simulink model "statcom_completed"  (Simulink 8.7)
settings: Solver=ode45  StartTime=0.0  StopTime=0.5  RelTol=1e-3
undefined symbols (not defined in the file): D11, Delta
libraries: powerlib x16, powerlib_extras x3
settings Model: Creator=CPLAB_9  LastModifiedBy=Shahrukh
settings DataIOCC: SignalLoggingSaveFormat=ModelDataLogs
settings OptimizationCC: ExpressionDepthLimit=2147483647
settings DebuggingCC: SolverPrmCheckMsg=warning  FcnCallInpInsideContextMsg=UseLocalSettings  StateNameClashWarn=warning
settings GRTTargetCC: CombineOutputUpdateFcns=off  GRTInterface=on

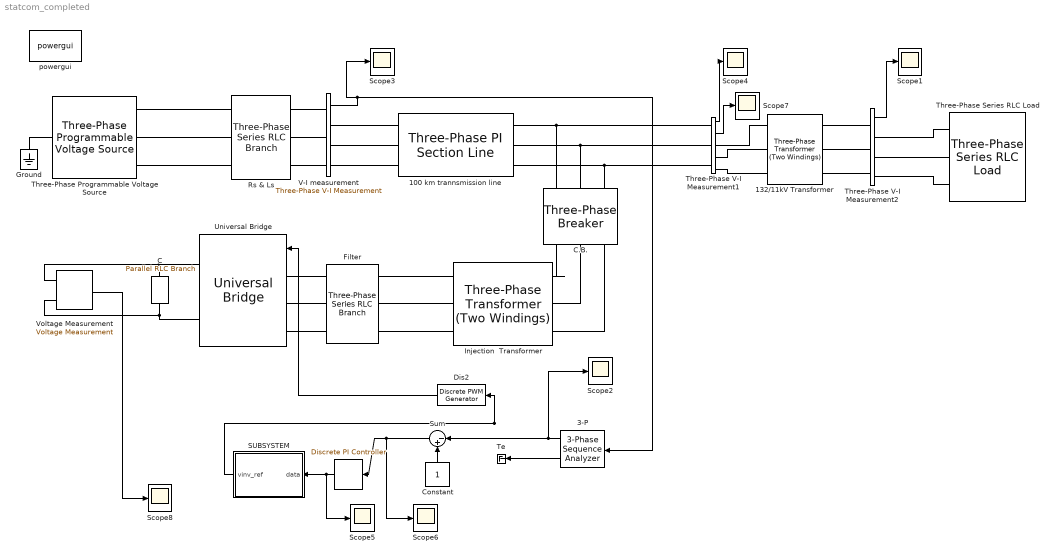
== system statcom_completed ==
  " " : powerlib_extras/Discrete  Control Blocks/Discrete PI Controller  Kp=0.5  Ki=500  Par_Limits=[1e6 -1e6]  Init=0  Ts=50e-6
  " 132/11kV Transformer" : powerlib/Elements/Three-Phase Transformer (Two Windings)  Winding1Connection=Delta (D11)  Winding2Connection=Delta (D11)  CoreType=Three single-phase transformers  SetSaturation=off  Hysteresis=off  DataFile='hysteresis'  SetInitialFlux=off  Measurements=None  UNITS=pu  NominalPower=[ 132e3 , 50 ]  Winding1="[ 132e3  , 0.01, 0.08 ]"  Winding2=[ 11e3 , 0.001, 0.008 ]  Rm=500  Lm=500  L0=0.5  Saturation=[ 0,0 ; 0.0024,1.2 ; 1.0,1.52 ]  InitialFluxes=[ 0.8 , -0.8 , 0.7 ]  MoreParameters=off  BreakLoop=off  DataType=off  TransfoNumber=1
  " Voltage Measurement" : powerlib/Measurements/Voltage Measurement  PhasorSimulation=off  OutputType=Complex  PSBequivalent=0
  "   C.B." : powerlib/Elements/Three-Phase Breaker  InitialState=open  SwitchA=on  SwitchB=on  SwitchC=on  SwitchTimes=[0.1 0.4]  External=off  BreakerResistance=0.01  SnubberResistance=1e5  SnubberCapacitance=inf  Measurements=Breaker voltages
  100 km trannsmission line : powerlib/Elements/Three-Phase PI Section Line  LConnTagsString=a|b|c  RConnTagsString=A|B|C  Frequency=50  Resistances=[ 0.00001 0.0001]  Inductances="[ 0.0000001e-3  0.0000001e-3]"  Capacitances=[0.00001e-9 0.000001e-9]  Length=100
  3-P : powerlib_extras/Measurements/3-Phase Sequence Analyzer  f1=50  n=1  seq=Positive
  C : powerlib/Elements/Parallel RLC Branch  LConnTagsString=a  RConnTagsString=__new0  BranchType=C  Resistance=[]  Inductance=[]  SetiL0=off  InitialCurrent=0  Capacitance=1000e-6  Setx0=off  InitialVoltage=600  Measurements=Branch voltage
  Constant : Constant
  Dis2 : powerlib_extras/Discrete  Control Blocks/Discrete PWM Generator  GeneratorMode="3-arm  bridge (6 pulses)"  Fc=5000  Ts=5e-6  Internal=off  mIndex=1  Freq=50  Phase=90
  Filter : powerlib/Elements/Three-Phase Series RLC Branch  LConnTagsString=A|B|C  RConnTagsString=A|B|C  BranchType=L  Resistance=0.001  Inductance=7.5  Capacitance=1.0  Measurements=Branch voltages
  Ground : powerlib/Elements/Ground  LConnTagsString=a
  Injection  Transformer : powerlib/Elements/Three-Phase Transformer (Two Windings)  Winding1Connection=Delta (D11)  Winding2Connection=Delta (D11)  CoreType=Three single-phase transformers  SetSaturation=off  Hysteresis=off  DataFile='hysteresis'  SetInitialFlux=off  Measurements=None  UNITS=pu  NominalPower=[ 132e3 , 50 ]  Winding1=[ 132e3 , 0.00002 , 0.00008 ]  Winding2=[ 11e3 , 0.00002 , 0.00008 ]  Rm=500  Lm=500  L0=0.5  Saturation=[ 0,0 ; 0.0024,1.2 ; 1.0,1.52 ]  InitialFluxes=[ 0.8 , -0.8 , 0.7 ]  MoreParameters=off  BreakLoop=off  DataType=off  TransfoNumber=1
  Rs & Ls : powerlib/Elements/Three-Phase Series RLC Branch  LConnTagsString=A|B|C  RConnTagsString=A|B|C  BranchType=RL  Resistance=0.02  Inductance=0.01  Capacitance=1.0  Measurements=Branch voltages
  SUBSYSTEM : Subsystem
  Scope{1..8} (8 alike) : Scope
  Sum : Sum  Inputs=|-+
  Te : Terminator
  Three-Phase Programmable Voltage Source : powerlib/Electrical Sources/Three-Phase Programmable Voltage Source  PositiveSequence="[132e3  0 50]"  VariationEntity=Amplitude  VariationType=Table of time-amplitude pairs  VariationTypeAlt=Step  VariationStep=0.5  VariationRate=10  VariationMagnitude=0.3  VariationFrequency=2  VariationTiming=[1 2]  VariationPhaseA=off  Amplitudes=[1 1.2 1 1]  TimeValues=[0 0.1 0.4 0.5]  HarmonicGeneration=off  HarmonicA=[3 0.2 -25 0]  HarmonicB=[2 0.15 35 2]  Timing="[0.05  3]"  BusType=swing  Pref=0  Qref=0  Qmin=-inf  Qmax=inf
  Three-Phase Series RLC Load : powerlib/Elements/Three-Phase Series RLC Load  LConnTagsString=A|B|C  Configuration=Y (grounded)  NominalVoltage=11e3  Vabc=[1e3 1e3 1e3]  Vabcp=[1e3 1e3 1e3]  NominalFrequency=50  UnbalancedPower=off  ActivePower=100e3  InductivePower=1000  CapacitivePower=1000  Pabc=[10e3 9e3 11e3]  QLabc=[100 90 110]  QCabc=[100 90 110]  Pabcp=[10e3 9e3 11e3]  QLabcp=[100 90 110]  QCabcp=[100 90 110]  Measurements=Branch voltages  LoadType=constant Z
  Three-Phase V-I Measurement1 : powerlib/Measurements/Three-Phase V-I Measurement  VoltageMeasurement=phase-to-ground  SetLabelV=off  LabelV=Vabc  Vpu=on  VpuLL=off  CurrentMeasurement=yes  SetLabelI=off  LabelI=Iabc  Ipu=off  Pbase=100e6  Vbase=132e3  OutputType=Complex  PhasorSimulation=off  PSBequivalent=0
  Three-Phase V-I Measurement2 : powerlib/Measurements/Three-Phase V-I Measurement  VoltageMeasurement=phase-to-phase  SetLabelV=off  LabelV=Vabc  Vpu=off  VpuLL=on  CurrentMeasurement=no  SetLabelI=off  LabelI=Iabc  Ipu=off  Pbase=100e6  Vbase=11e3  OutputType=Complex  PhasorSimulation=off  PSBequivalent=0
  Universal Bridge : powerlib/Power Electronics/Universal Bridge  Arms=3  SnubberResistance=1e5  SnubberCapacitance=inf  Device=IGBT / Diodes  Ron=1e-3  Lon=0  ForwardVoltages="[  0  0  ]"  ForwardVoltage=0  GTOparameters=[ 10e-6 , 20e-6 ]  IGBTparameters=[ 1e-6 , 2e-6 ]  Measurements=None  Measurements_2=None  converterType=Rectifier
      link override Uswitch: GotoTag=tp182559
  V-I measurement : powerlib/Measurements/Three-Phase V-I Measurement  VoltageMeasurement=phase-to-ground  SetLabelV=off  LabelV=Vabc  Vpu=on  VpuLL=off  CurrentMeasurement=no  SetLabelI=off  LabelI=Iabc  Ipu=off  Pbase=100e6  Vbase=132e3  OutputType=Complex  PhasorSimulation=off  PSBequivalent=0
  powergui : powerlib/powergui  Priority=1  SimulationMode=Discrete  SolverType=Tustin/Backward Euler (TBE)  SampleTime=50e-6  frequency=60  SPID=off  DisableSnubberDevices=off  DisableRonSwitches=off  DisableVfSwitches=off  SwTol=0  DisplayEquations=off  Interpol=off  ExternalGateDelay=off  methode=off  Ts=10  FunctionMessages=off  echomessages=off  HookPort=off  EnableUseOfTLC=off  x0status=blocks  frequencyindice=50  Pbase=100e6  ErrMax=1e-4  Iterations=50  UnitsV=kV  UnitsW=MW  buscounter=0  RestoreLinks=warning  ResistiveCurrentMeasurement=off  Frange=[0:2:500]  Ylog=off  Xlog=on  ShowGrid=off  save=off  variable=ZData  structure=ScopeData2  ZoomFFT=off  StartTime=0.001  cycles=3  DisplayStyle=1  fundamental=50  FreqAxis=on  MaxFrequency=50  frequencyindicesteady=1  RmsSteady=1  display=off
  wires:
  3-P/2 -> Te/1
  3-P/1 -> Sum/1, Scope2/1
  Constant/1 -> Sum/2
  Sum/1 -> " "/1, Scope6/1
  " "/1 -> SUBSYSTEM/1(data), Scope5/1
  V-I measurement/1 -> Scope3/1, 3-P/1
  Three-Phase V-I Measurement1/1 -> Scope4/1
  Three-Phase V-I Measurement2/1 -> Scope1/1
  SUBSYSTEM/1(vinv_ref) -> Dis2/1
  Dis2/1 -> Universal Bridge/1
  " Voltage Measurement"/1 -> Scope8/1
  Three-Phase V-I Measurement1/2 -> Scope7/1
  connections:
  Three-Phase Programmable Voltage Source/RConn1 -- Rs & Ls/LConn1
  Three-Phase Programmable Voltage Source/RConn2 -- Rs & Ls/LConn2
  Three-Phase Programmable Voltage Source/RConn3 -- Rs & Ls/LConn3
  Rs & Ls/RConn1 -- V-I measurement/LConn1
  Rs & Ls/RConn2 -- V-I measurement/LConn2
  Rs & Ls/RConn3 -- V-I measurement/LConn3
  Ground/LConn1 -- Three-Phase Programmable Voltage Source/LConn1
  100 km trannsmission line/RConn1 -- "   C.B."/RConn1 -- Three-Phase V-I Measurement1/LConn1
  100 km trannsmission line/RConn2 -- "   C.B."/RConn2 -- Three-Phase V-I Measurement1/LConn2
  100 km trannsmission line/RConn3 -- "   C.B."/RConn3 -- Three-Phase V-I Measurement1/LConn3
  Universal Bridge/RConn1 -- " Voltage Measurement"/LConn1 -- C/LConn1
  Universal Bridge/LConn1 -- Filter/RConn1
  Universal Bridge/LConn2 -- Filter/RConn2
  Universal Bridge/LConn3 -- Filter/RConn3
  Universal Bridge/RConn2 -- " Voltage Measurement"/LConn2 -- C/RConn1
  Three-Phase V-I Measurement1/RConn1 -- " 132/11kV Transformer"/LConn1
  Three-Phase V-I Measurement1/RConn2 -- " 132/11kV Transformer"/LConn2
  Three-Phase V-I Measurement1/RConn3 -- " 132/11kV Transformer"/LConn3
  Three-Phase Series RLC Load/LConn2 -- Three-Phase V-I Measurement2/RConn2
  " 132/11kV Transformer"/RConn3 -- Three-Phase V-I Measurement2/LConn3
  Three-Phase V-I Measurement2/LConn2 -- " 132/11kV Transformer"/RConn2
  " 132/11kV Transformer"/RConn1 -- Three-Phase V-I Measurement2/LConn1
  Three-Phase V-I Measurement2/RConn3 -- Three-Phase Series RLC Load/LConn3
  Three-Phase V-I Measurement2/RConn1 -- Three-Phase Series RLC Load/LConn1
  Injection  Transformer/RConn2 -- "   C.B."/LConn2
  Injection  Transformer/RConn1 -- "   C.B."/LConn1
  Injection  Transformer/RConn3 -- "   C.B."/LConn3
  Filter/LConn1 -- Injection  Transformer/LConn1
  Filter/LConn3 -- Injection  Transformer/LConn3
  Injection  Transformer/LConn2 -- Filter/LConn2
  100 km trannsmission line/LConn1 -- V-I measurement/RConn1
  100 km trannsmission line/LConn2 -- V-I measurement/RConn2
  100 km trannsmission line/LConn3 -- V-I measurement/RConn3

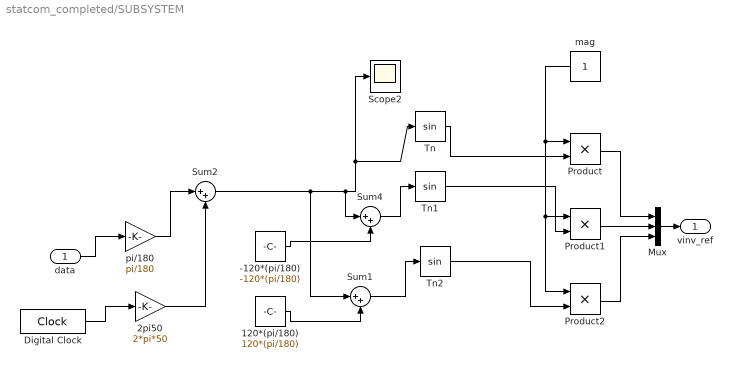
== system statcom_completed/SUBSYSTEM ==
  data : Inport
  -120*(pi/180) : Constant  Value=-120*(pi/180)
  120*(pi/180) : Constant  Value=120*(pi/180)
  2pi50 : Gain  Gain=2*pi*50
  Digital Clock : DigitalClock  SampleTime=5e-6
  Mux : Mux  Inputs=3
  Product : Product  RndMeth=Zero
  Product1 : Product  RndMeth=Zero
  Product2 : Product  RndMeth=Zero
  Scope2 : Scope
  Sum1 : Sum  Inputs=|++
  Sum2 : Sum  Inputs=|++
  Sum4 : Sum  Inputs=|++
  Tn : Trigonometry  SampleTime=1
  Tn1 : Trigonometry
  Tn2 : Trigonometry
  mag : Constant
  pi/180 : Gain  Gain=pi/180
  vinv_ref : Outport
  wires:
  Tn1/1 -> Product1/2
  Tn/1 -> Product/2
  Mux/1 -> vinv_ref/1
  Product2/1 -> Mux/3
  Product1/1 -> Mux/2
  Product/1 -> Mux/1
  data/1 -> pi/180/1
  Digital Clock/1 -> 2pi50/1
  2pi50/1 -> Sum2/2
  pi/180/1 -> Sum2/1
  120*(pi/180)/1 -> Sum1/2
  Sum1/1 -> Tn2/1
  -120*(pi/180)/1 -> Sum4/2
  Sum4/1 -> Tn1/1
  Sum2/1 -> Sum1/1, Tn/1, Scope2/1, Sum4/1
  Tn2/1 -> Product2/2
  mag/1 -> Product/1, Product1/1, Product2/1
